simulink model "Lyapunov_Control"  (R2015b)
settings: Solver=ode8  StartTime=0  StopTime=26  FixedStep=0.1  RelTol=1e-3
values from neighbouring files (symbols this model uses):
  Ktheta = 5    [init.m]
  Kx = 5    [init.m]
  Ky = 5    [init.m]
  L = 0.13    [init.m]
  r = 0.1    [init.m]
  R = 2    [init.m]
  Theta0 = pi    (= 3.14159265359)    [init.m]
  wd = 0.5    [init.m]
  X0 = 2.3    [init.m]
  Y0 = 0    [init.m]
undefined symbols (not defined in the file): alpha
libraries: simulink x2
settings Model: Creator=GANESH  LastModifiedBy=GANESH

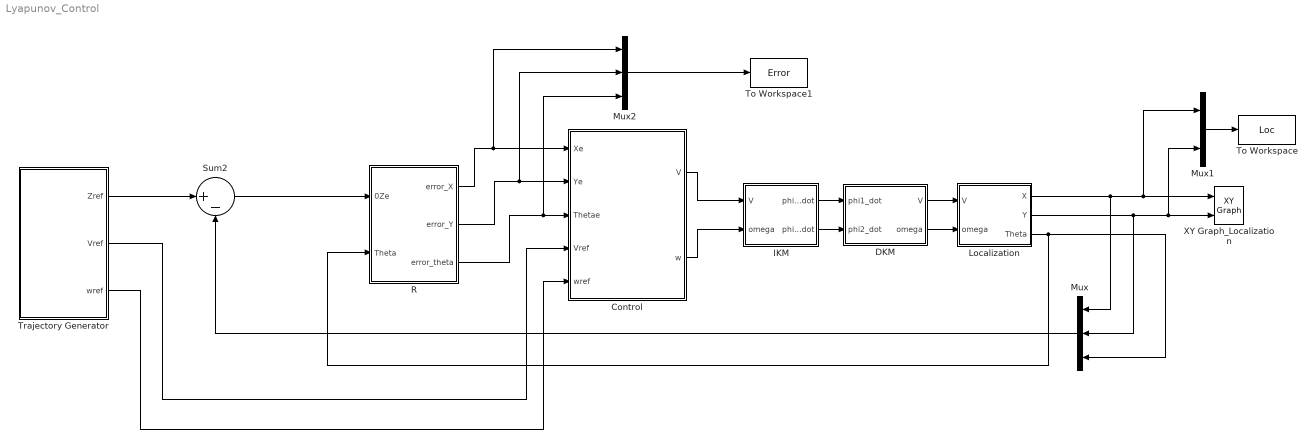
== system Lyapunov_Control ==
  "Control " : Subsystem
  DKM : Subsystem  mask{r=r, L=L}
      mask prompts: r "Radius of the wheel"; L "Half of the wheelbase"
  IKM : Subsystem  mask{r=(1+alpha)*r, L=(1+alpha)*L}
      mask prompts: r "Radius of wheel (estimated)"; L "Half of wheelbase (estimated)"
  Localization : Subsystem
  Mux : Mux  Inputs=3
  Mux1 : Mux  Inputs=2
  Mux2 : Mux  Inputs=3
  R : Subsystem
  Sum2 : Sum  Inputs=|+-
  To Workspace : ToWorkspace  VariableName=Loc  SaveFormat=Timeseries  SampleTime=-1
  To Workspace1 : ToWorkspace  VariableName=Error  SaveFormat=Timeseries  SampleTime=-1
  Trajectory Generator : Subsystem  mask{R=R, wd=wd}
      mask prompts: R "Radius of Circular Trajectory"; wd "Desired Angular Velocity"
  XY Graph_Localization : simulink/Sinks/XY Graph  xmin=-5  xmax=5  ymin=-5  ymax=5  st=-1
  wires:
  IKM/1(phi1_dot) -> DKM/1(phi1_dot)
  IKM/2(phi2_dot) -> DKM/2(phi2_dot)
  "Control "/1(V) -> IKM/1(V)
  "Control "/2(w) -> IKM/2(omega)
  DKM/1(V) -> Localization/1(V)
  DKM/2(omega) -> Localization/2(omega)
  R/1(error_X) -> Mux2/1, "Control "/1(Xe)
  R/2(error_Y) -> Mux2/2, "Control "/2(Ye)
  R/3(error_theta) -> Mux2/3, "Control "/3(Thetae)
  Localization/2(Y) -> Mux/2, Mux1/2, XY Graph_Localization/2
  Localization/1(X) -> Mux1/1, XY Graph_Localization/1, Mux/1
  Localization/3(Theta) -> Mux/3, R/2(Theta)
  Trajectory Generator/1(Zref) -> Sum2/1
  Sum2/1 -> R/1(0Ze)
  Mux/1 -> Sum2/2
  Trajectory Generator/2(Vref) -> "Control "/4("Vref ")
  Trajectory Generator/3(wref) -> "Control "/5(wref)
  Mux1/1 -> To Workspace/1
  Mux2/1 -> To Workspace1/1

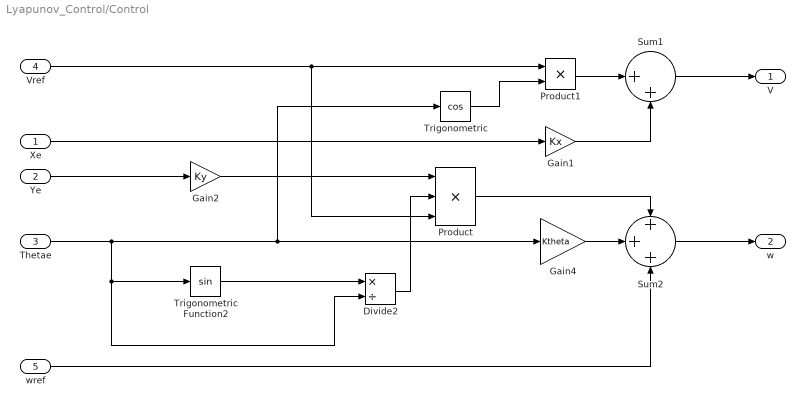
== system Lyapunov_Control/Control  ==
  Xe : Inport
  Ye : Inport  Port=2
  Thetae : Inport  Port=3
  "Vref " : Inport  Port=4
  wref : Inport  Port=5
  Divide2 : Product  Inputs=*/
  Gain1 : Gain  Gain=Kx
  Gain2 : Gain  Gain=Ky
  Gain4 : Gain  Gain=Ktheta
  Product : Product  Inputs=3
  Product1 : Product
  Sum1 : Sum  Inputs=|++
  Sum2 : Sum  Inputs=+++
  "Trigonometric " : Trigonometry  Operator=cos
  Trigonometric Function2 : Trigonometry
  V : Outport
  w : Outport  Port=2
  wires:
  "Trigonometric "/1 -> Product1/2
  Sum1/1 -> V/1
  Xe/1 -> Gain1/1
  Thetae/1 -> "Trigonometric "/1, Gain4/1, Trigonometric Function2/1, Divide2/2
  Sum2/1 -> w/1
  Product/1 -> Sum2/1
  Gain4/1 -> Sum2/2
  Product1/1 -> Sum1/1
  Gain1/1 -> Sum1/2
  "Vref "/1 -> Product1/1, Product/3
  wref/1 -> Sum2/3
  Trigonometric Function2/1 -> Divide2/1
  Divide2/1 -> Product/2
  Ye/1 -> Gain2/1
  Gain2/1 -> Product/1

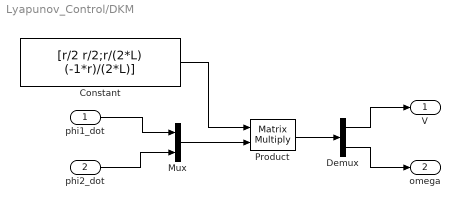
== system Lyapunov_Control/DKM ==
  phi1_dot : Inport
  phi2_dot : Inport  Port=2
  Constant : Constant  Value=[r/2 r/2;r/(2*L) (-1*r)/(2*L)]
  Demux : Demux  Outputs=2
  Mux : Mux  Inputs=2
  Product : Product  Multiplication=Matrix(*)
  V : Outport
  omega : Outport  Port=2
  wires:
  Product/1 -> Demux/1
  phi1_dot/1 -> Mux/1
  Demux/1 -> V/1
  phi2_dot/1 -> Mux/2
  Constant/1 -> Product/1
  Demux/2 -> omega/1
  Mux/1 -> Product/2

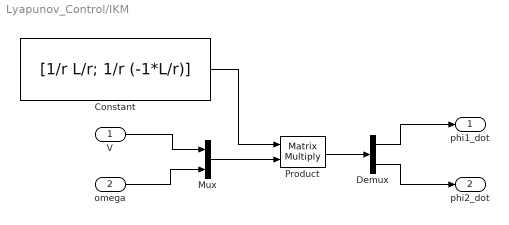
== system Lyapunov_Control/IKM ==
  V : Inport
  omega : Inport  Port=2
  Constant : Constant  Value=[1/r L/r; 1/r (-1*L/r)]
  Demux : Demux  Outputs=2
  Mux : Mux  Inputs=2
  Product : Product  Multiplication=Matrix(*)
  phi1_dot : Outport
  phi2_dot : Outport  Port=2
  wires:
  Product/1 -> Demux/1
  V/1 -> Mux/1
  Demux/1 -> phi1_dot/1
  omega/1 -> Mux/2
  Constant/1 -> Product/1
  Mux/1 -> Product/2
  Demux/2 -> phi2_dot/1

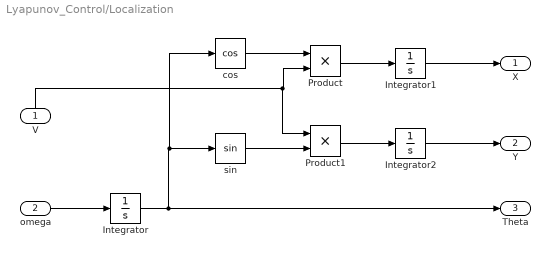
== system Lyapunov_Control/Localization ==
  V : Inport
  omega : Inport  Port=2
  Integrator : Integrator  InitialCondition=Theta0
  Integrator1 : Integrator  InitialCondition=X0
  Integrator2 : Integrator  InitialCondition=Y0
  Product : Product
  Product1 : Product
  cos : Trigonometry  Operator=cos
  sin : Trigonometry
  X : Outport
  Y : Outport  Port=2
  Theta : Outport  Port=3
  wires:
  Integrator/1 -> Theta/1, cos/1, sin/1
  V/1 -> Product1/1, Product/2
  omega/1 -> Integrator/1
  cos/1 -> Product/1
  sin/1 -> Product1/2
  Integrator1/1 -> X/1
  Product1/1 -> Integrator2/1
  Integrator2/1 -> Y/1
  Product/1 -> Integrator1/1

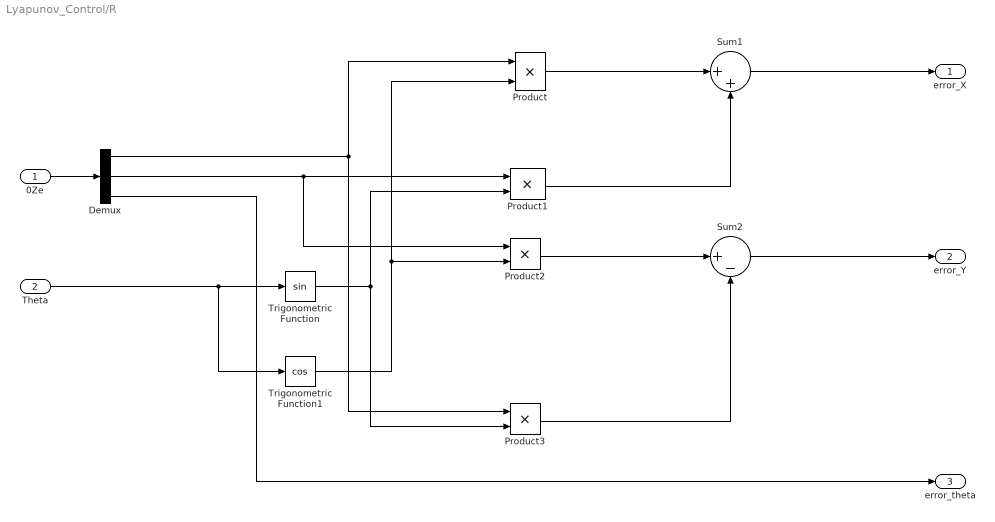
== system Lyapunov_Control/R ==
  0Ze : Inport
  Theta : Inport  Port=2
  Demux : Demux  Outputs=3
  Product{,1..3} (4 alike) : Product
  Sum1 : Sum  Inputs=|++
  Sum2 : Sum  Inputs=|+-
  Trigonometric Function : Trigonometry
  Trigonometric Function1 : Trigonometry  Operator=cos
  error_X : Outport
  error_Y : Outport  Port=2
  error_theta : Outport  Port=3
  wires:
  Theta/1 -> Trigonometric Function/1, Trigonometric Function1/1
  Sum1/1 -> error_X/1
  Sum2/1 -> error_Y/1
  Demux/1 -> Product/1, Product3/1
  Trigonometric Function1/1 -> Product2/2, Product/2
  Product/1 -> Sum1/1
  Demux/2 -> Product1/1, Product2/1
  Trigonometric Function/1 -> Product1/2, Product3/2
  Product1/1 -> Sum1/2
  Product2/1 -> Sum2/1
  Product3/1 -> Sum2/2
  Demux/3 -> error_theta/1
  0Ze/1 -> Demux/1

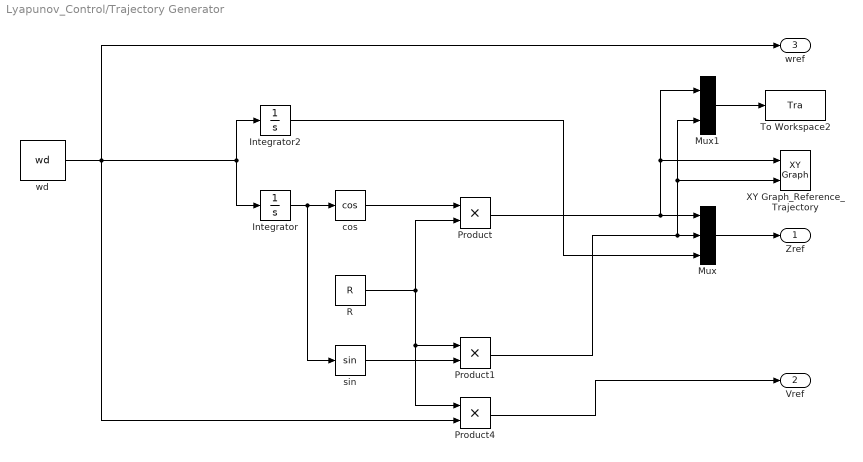
== system Lyapunov_Control/Trajectory Generator ==
  Integrator : Integrator
  Integrator2 : Integrator  InitialCondition=pi/2
  Mux : Mux  Inputs=3
  Mux1 : Mux  Inputs=2
  Product : Product
  Product1 : Product
  Product4 : Product
  R : Constant  Value=R
  To Workspace2 : ToWorkspace  VariableName=Tra  SaveFormat=Timeseries  SampleTime=-1
  XY Graph_Reference_Trajectory : simulink/Sinks/XY Graph  xmin=-5  xmax=5  ymin=-5  ymax=5  st=-1
  cos : Trigonometry  Operator=cos
  sin : Trigonometry
  wd : Constant  Value=wd
  Zref : Outport
  Vref : Outport  Port=2
  wref : Outport  Port=3
  wires:
  R/1 -> Product4/1, Product1/1, Product/2
  Product1/1 -> Mux1/2, XY Graph_Reference_Trajectory/2, Mux/2
  Product/1 -> Mux1/1, XY Graph_Reference_Trajectory/1, Mux/1
  wd/1 -> Integrator2/1, Integrator/1, wref/1, Product4/2
  Integrator/1 -> cos/1, sin/1
  Product4/1 -> Vref/1
  cos/1 -> Product/1
  sin/1 -> Product1/2
  Integrator2/1 -> Mux/3
  Mux/1 -> Zref/1
  Mux1/1 -> To Workspace2/1
